simulink model "scattering_pos_pos"  (R2022b)
settings: Solver=VariableStepAuto  StartTime=0.0  StopTime=10.0  RelTol=1e-3
values from neighbouring files (symbols this model uses):
  A = 2    [scattering_params.m]    (also in scattering_params_force_pos.m = 3; scattering_params_pos_pos.m = 1)
  b = 1    [scattering_params.m]    (also in scattering_params_force_pos.m = 40; scattering_params_pos_pos.m = 100)
  Be = 100    [scattering_params.m]    (also in scattering_params_force_pos.m; scattering_params_pos_pos.m)
  Bh = 1.5    [scattering_params.m]    (also in scattering_params_force_pos.m = 1; scattering_params_pos_pos.m = 1)
  Bm = 20*0.8    (= 16)    [scattering_params.m]
  Bs = 80    [scattering_params.m]    (also in scattering_params_force_pos.m = 10)
  Dh = 0.1    [scattering_params.m]    (also in scattering_params_force_pos.m = 16; scattering_params_pos_pos.m = 16)
  Dm = 0    [scattering_params.m]    (also in scattering_params_force_pos.m; scattering_params_pos_pos.m)
  Ds = 0    [scattering_params.m]    (also in scattering_params_force_pos.m; scattering_params_pos_pos.m)
  Fc = 1    [scattering_params.m]    (also in scattering_params_force_pos.m = 0.25; scattering_params_pos_pos.m = 0.25)
  Flp = 5    [scattering_params.m]    (also in scattering_params_force_pos.m = 0.5; scattering_params_pos_pos.m = 0.5)
  Jh = 1    [scattering_params.m]    (also in scattering_params_force_pos.m; scattering_params_pos_pos.m)
  Ke = 200    [scattering_params.m]    (also in scattering_params_force_pos.m; scattering_params_pos_pos.m)
  Km = 10*1    (= 10)    [scattering_params.m]
  Ks = 100    [scattering_params.m]    (also in scattering_params_force_pos.m)
  Mm = 0.5    [scattering_params.m]    (also in scattering_params_force_pos.m; scattering_params_pos_pos.m)
  Ms = 2    [scattering_params.m]    (also in scattering_params_force_pos.m; scattering_params_pos_pos.m)
  Ph = 10    [scattering_params.m]    (also in scattering_params_force_pos.m; scattering_params_pos_pos.m)
  time_delay = 0    [scattering_params.m]
  xe = 5    [scattering_params.m]    (also in scattering_params_force_pos.m = 2; scattering_params_pos_pos.m = 2)
settings Model: Creator=Manu  LastModifiedBy=Manu

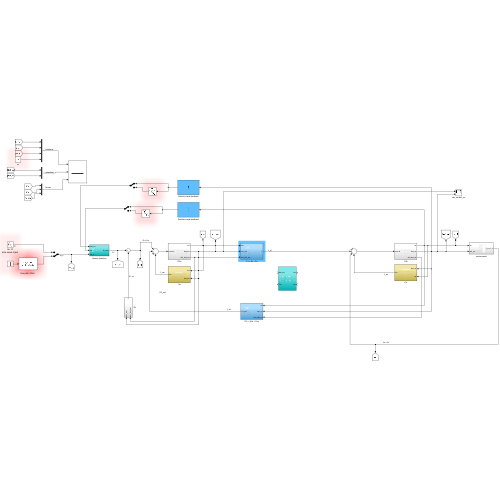
[thumbnail: Simulink's stored preview of the top-level diagram]
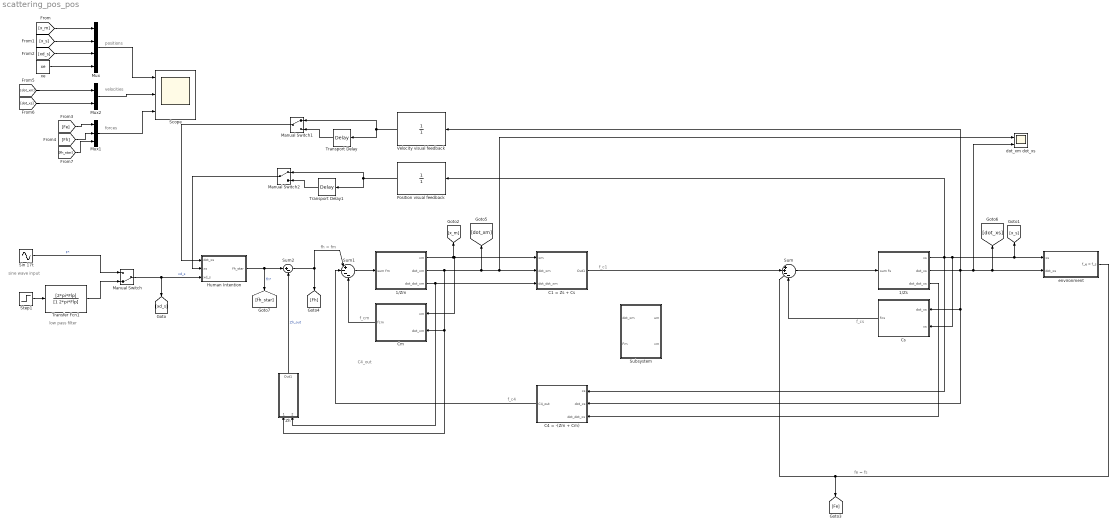
== system scattering_pos_pos ==
  note: positions
  note: fe = fs
  note: C4_out
  note: f_cm
  note: fh = fm
  note: sine wave input
  note: low pass filter
  note: f_cs
  note: forces
  note: velocities
  note: f_c4
  note: f_c1
  1/Zm : Subsystem
  1/Zs : Subsystem
  C1 = Zs + Cs : Subsystem
  C4 = -(Zm + Cm) : Subsystem
  Cm : Subsystem
  Cs : Subsystem
  Human Intention : Subsystem
  Manual Switch : ManualSwitch  CurrentSetting=0
  Manual Switch1 : ManualSwitch
  Manual Switch2 : ManualSwitch
  Mux : Mux
  Mux1 : Mux  Inputs=3
  Mux2 : Mux  Inputs=2
  Position visual feedback : TransferFcn  Denominator=[1]
  Scope : Scope  NumInputPorts=3
  Sin 17t : Sin  Amplitude=A  Frequency=2*pi*Fc  SampleTime=0
  Step1 : Step  Time=0.5  After=A  SampleTime=0
  Subsystem : Subsystem
      settings: PortSchema="{\"entries\":[{\"content\":{\"sides\":[{\"content\":{\"connectorIds\":[\"In1\",\"Out2\"]},\"type\":\"ConnectorPlacement.EquallySpacedRectSide\",\"uuid\":\"82be490b-f4e1-4469-8bd6-488a0e070f91\"},{\"content\":{\"connectorIds\":[\"Out1\",\"In2\"],\"side\":\"RIGHT\"},\"type\":\"ConnectorPlacement.EquallySpacedRectSide\",\"uuid\":\"c4a13bf6-21c5-475e-be70-cb3636e820b8\"},{\"content\":{\"connectorIds\":[],\"side\":\"TOP\"},\"type\":\"ConnectorPlacement.EquallySpacedRectSide\",\"uuid\":\"239945ea-98d9-43ca-9337-d0acd489fa2c\"},{\"content\":{\"connectorIds\":[],\"side\":\"BOTTOM\"},\"type\":\"ConnectorPlacement.EquallySpacedRectSide\",\"uuid\":\"d302d15a-ee16-4e35-85d1-74674ea2a331\"},{\"content\":{\"connectorIds\":[],\"side\":\"HIDDEN\"},\"type\":\"ConnectorPlacement.EquallySpacedRectSide\",\"uuid\":\"ab55d6c9-2d6b-496a-b62d-f74546630c92\"}]},\"type\":\"ConnectorPlacement.EquallySpacedConnector\",\"uuid\":\"f2ee4140-76ed-4153-9f7f-3580e67d072a\"}],\"packageUris\":[\"http://schema.mathworks.com/mf0/Connector/R2020b\"],\"version\":\"1.0\"}"
  Sum : Sum  Inputs=|++--
  Sum1 : Sum  Inputs=|+---
  Sum2 : Sum  Inputs=|+-
  Transfer Fcn1 : TransferFcn  Numerator=[2*pi*Flp]  Denominator=[1 2*pi*Flp]
  Transport Delay : TransportDelay  DelayTime=time_delay
  Transport Delay1 : TransportDelay  DelayTime=time_delay
  Velocity visual feedback : TransferFcn  Denominator=[1]
  Zh : Subsystem
  dot_xm dot_xs : Scope  NumInputPorts=2
  environment : Subsystem
  xe : Constant  Value=xe
  wires:
  1/Zm/2(dot_xm) -> C1 = Zs + Cs/2(dot_xm), dot_xm dot_xs/1, [dot_xm], Cm/2(dot_xm), Zh/1(dot_xm)
  1/Zm/1(xm) -> C1 = Zs + Cs/1(xm), Cm/1(xm), [x_m]
  Manual Switch/1 -> [xd_s], Human Intention/3(xd_s)  "xd_s"
  Zh/1(Out1) -> Sum2/2  "Zh_out"
  Sin 17t/1 -> Manual Switch/1  "F*"
  1/Zm/3(dot_dot_xm) -> C1 = Zs + Cs/3(dot_dot_xm), Zh/2(dot_dot_xm)
  Human Intention/1(fh_star) -> Sum2/1, [fh_star]  "fh*"
  Transfer Fcn1/1 -> Manual Switch/2
  Step1/1 -> Transfer Fcn1/1
  Sum2/1 -> Sum1/1, [Fh]
  Sum1/1 -> 1/Zm/1(sum fm)
  C4 = -(Zm + Cm)/1(C4_out) -> Sum1/2
  C1 = Zs + Cs/1(Out1) -> Sum/2
  Cs/1(fcs) -> Sum/4
  Sum/1 -> 1/Zs/1(sum fs)
  1/Zs/2(dot_xs) -> Velocity visual feedback/1, C4 = -(Zm + Cm)/2(dot_xs), Cs/1(dot_xs), dot_xm dot_xs/2, [dot_xs], environment/2(dot_xs)
  1/Zs/1(xs) -> C4 = -(Zm + Cm)/1(xs), Cs/2(xs), [x_s], environment/1(xs), Position visual feedback/1
  1/Zs/3(dot_dot_xs) -> C4 = -(Zm + Cm)/3(dot_dot_xs)
  environment/1(f_e = f_s) -> Sum/3, [Fe]
  Cm/1(fcm) -> Sum1/4
  Mux/1 -> Scope/1
  [x_s] -> Mux/2
  [xd_s] -> Mux/3
  xe/1 -> Mux/4
  [x_m] -> Mux/1
  Mux1/1 -> Scope/3
  [Fe] -> Mux1/1
  [Fh] -> Mux1/2
  [dot_xs] -> Mux2/2
  [dot_xm] -> Mux2/1
  Mux2/1 -> Scope/2
  [fh_star] -> Mux1/3
  Velocity visual feedback/1 -> Transport Delay/1, Manual Switch1/1
  Transport Delay/1 -> Manual Switch1/2
  Manual Switch1/1 -> Human Intention/1(dot_xs)
  Transport Delay1/1 -> Manual Switch2/2
  Position visual feedback/1 -> Transport Delay1/1, Manual Switch2/1
  Manual Switch2/1 -> Human Intention/2(xs)

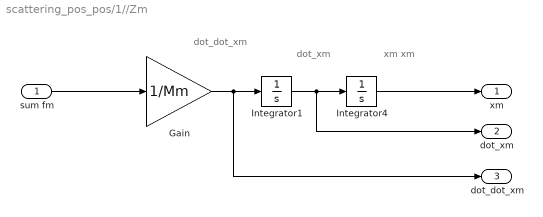
== system scattering_pos_pos/1//Zm ==
  note: dot_dot_xm
  note: dot_xm
  note: xm
      | xm
  sum fm : Inport
  Gain : Gain  Gain=1/Mm
  Integrator1 : Integrator
  Integrator4 : Integrator
  xm : Outport
  dot_xm : Outport  Port=2
  dot_dot_xm : Outport  Port=3
  wires:
  sum fm/1 -> Gain/1
  Gain/1 -> dot_dot_xm/1, Integrator1/1
  Integrator4/1 -> xm/1
  Integrator1/1 -> dot_xm/1, Integrator4/1

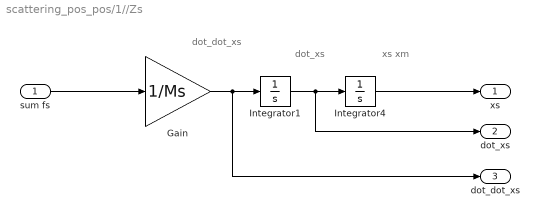
== system scattering_pos_pos/1//Zs ==
  note: dot_dot_xs
  note: dot_xs
  note: xs
      | xm
  sum fs : Inport
  Gain : Gain  Gain=1/Ms
  Integrator1 : Integrator
  Integrator4 : Integrator
  xs : Outport
  dot_xs : Outport  Port=2
  dot_dot_xs : Outport  Port=3
  wires:
  sum fs/1 -> Gain/1
  Gain/1 -> dot_dot_xs/1, Integrator1/1
  Integrator4/1 -> xs/1
  Integrator1/1 -> dot_xs/1, Integrator4/1

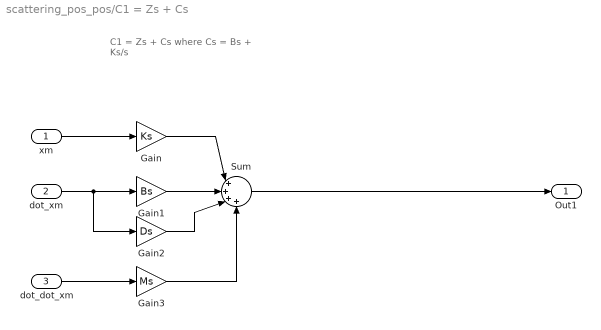
== system scattering_pos_pos/C1 = Zs + Cs ==
  note: C1 = Zs + Cs
      | where
      | Cs = Bs + Ks/s
  xm : Inport
  dot_xm : Inport  Port=2
  dot_dot_xm : Inport  Port=3
  Gain : Gain  Gain=Ks
  Gain1 : Gain  Gain=Bs
  Gain2 : Gain  Gain=Ds
  Gain3 : Gain  Gain=Ms
  Sum : Sum  Inputs=|++++
  Out1 : Outport
  wires:
  xm/1 -> Gain/1
  Gain/1 -> Sum/1
  dot_xm/1 -> Gain2/1, Gain1/1
  Gain1/1 -> Sum/2
  Gain2/1 -> Sum/3
  dot_dot_xm/1 -> Gain3/1
  Gain3/1 -> Sum/4
  Sum/1 -> Out1/1

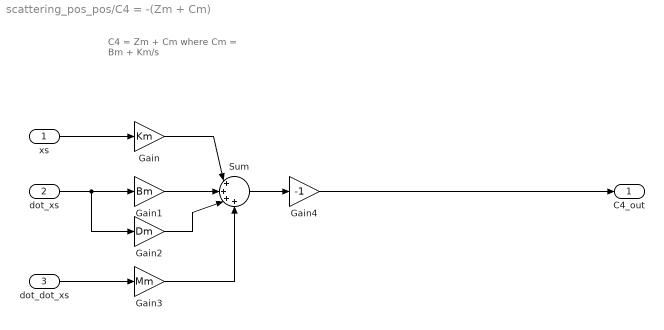
== system scattering_pos_pos/C4 = -(Zm + Cm) ==
  note: C4 = Zm + Cm
      | where
      | Cm = Bm + Km/s
  xs : Inport
  dot_xs : Inport  Port=2
  dot_dot_xs : Inport  Port=3
  Gain : Gain  Gain=Km
  Gain1 : Gain  Gain=Bm
  Gain2 : Gain  Gain=Dm
  Gain3 : Gain  Gain=Mm
  Gain4 : Gain  Gain=-1
  Sum : Sum  Inputs=|++++
  C4_out : Outport
  wires:
  xs/1 -> Gain/1
  Gain/1 -> Sum/1
  dot_xs/1 -> Gain2/1, Gain1/1
  Gain1/1 -> Sum/2
  Gain2/1 -> Sum/3
  dot_dot_xs/1 -> Gain3/1
  Gain3/1 -> Sum/4
  Sum/1 -> Gain4/1
  Gain4/1 -> C4_out/1

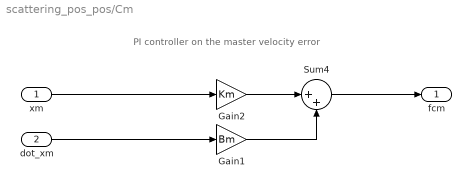
== system scattering_pos_pos/Cm ==
  note: PI controller on the master velocity error
  xm : Inport
  dot_xm : Inport  Port=2
  Gain1 : Gain  Gain=Bm
  Gain2 : Gain  Gain=Km
  Sum4 : Sum  Inputs=|++
  fcm : Outport
  wires:
  Sum4/1 -> fcm/1
  xm/1 -> Gain2/1
  Gain2/1 -> Sum4/1
  dot_xm/1 -> Gain1/1
  Gain1/1 -> Sum4/2

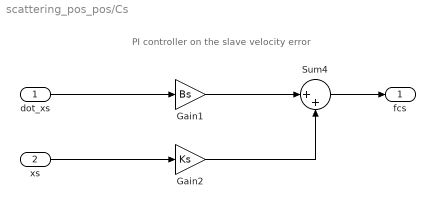
== system scattering_pos_pos/Cs ==
  note: PI controller on the slave velocity error
  dot_xs : Inport
  xs : Inport  Port=2
  Gain1 : Gain  Gain=Bs
  Gain2 : Gain  Gain=Ks
  Sum4 : Sum  Inputs=|++
  fcs : Outport
  wires:
  Sum4/1 -> fcs/1
  xs/1 -> Gain2/1
  Gain2/1 -> Sum4/2
  dot_xs/1 -> Gain1/1
  Gain1/1 -> Sum4/1

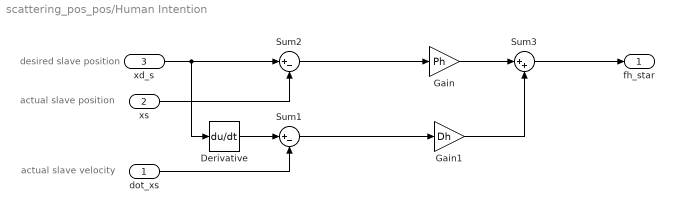
== system scattering_pos_pos/Human Intention ==
  note: actual slave velocity
  note: actual slave position
  note: desired slave position
  dot_xs : Inport
  xs : Inport  Port=2
  xd_s : Inport  Port=3
  Derivative : Derivative
  Gain : Gain  Gain=Ph
  Gain1 : Gain  Gain=Dh
  Sum1 : Sum  Inputs=|+-
  Sum2 : Sum  Inputs=|+-
  Sum3 : Sum  Inputs=|++
  fh_star : Outport
  wires:
  xs/1 -> Sum2/2
  dot_xs/1 -> Sum1/2
  Sum2/1 -> Gain/1
  Sum1/1 -> Gain1/1
  Gain1/1 -> Sum3/2
  Gain/1 -> Sum3/1
  Sum3/1 -> fh_star/1
  xd_s/1 -> Derivative/1, Sum2/1
  Derivative/1 -> Sum1/1

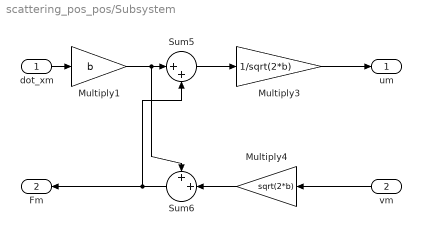
== system scattering_pos_pos/Subsystem ==
  dot_xm : Inport
  vm : Inport  Port=2
  Multiply1 : Gain  Gain=b
  Multiply3 : Gain  Gain=1/sqrt(2*b)
  Multiply4 : Gain  Gain=sqrt(2*b)
  Sum5 : Sum  Inputs=|++
  Sum6 : Sum  Inputs=++|
  um : Outport
  Fm : Outport  Port=2
  wires:
  Sum6/1 -> Fm/1, Sum5/2
  Multiply1/1 -> Sum6/1, Sum5/1
  Sum5/1 -> Multiply3/1
  Multiply4/1 -> Sum6/2
  vm/1 -> Multiply4/1
  Multiply3/1 -> um/1
  dot_xm/1 -> Multiply1/1

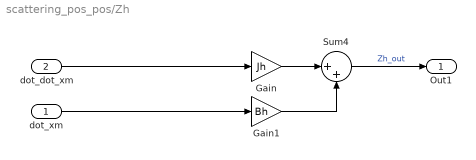
== system scattering_pos_pos/Zh ==
  dot_xm : Inport
  dot_dot_xm : Inport  Port=2
  Gain : Gain  Gain=Jh
  Gain1 : Gain  Gain=Bh
  Sum4 : Sum  Inputs=|++
  Out1 : Outport
  wires:
  dot_dot_xm/1 -> Gain/1
  Gain1/1 -> Sum4/2
  Gain/1 -> Sum4/1
  Sum4/1 -> Out1/1  "Zh_out"
  dot_xm/1 -> Gain1/1

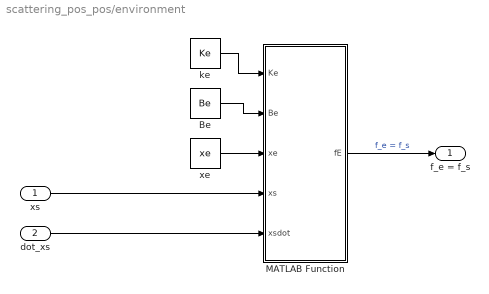
== system scattering_pos_pos/environment ==
  xs : Inport
  dot_xs : Inport  Port=2
  Be : Constant  Value=Be
  MATLAB Function : MATLAB Function  TreatAsAtomicUnit=on
  ke : Constant  Value=Ke
  xe : Constant  Value=xe
  f_e = f_s : Outport
  wires:
  MATLAB Function/1(fE) -> f_e = f_s/1  "f_e = f_s"
  xs/1 -> MATLAB Function/4(xs)
  xe/1 -> MATLAB Function/3(xe)
  dot_xs/1 -> MATLAB Function/5(xsdot)
  ke/1 -> MATLAB Function/1(Ke)
  Be/1 -> MATLAB Function/2(Be)

== matlab function scattering_pos_pos/environment/MATLAB Function ==
  data: Ke input; fE output; Be input; xe input; xs input; xsdot input
function fE = environment(Ke, Be, xe, xs, xsdot)
    if xs > xe
        fE = Ke * (xs - xe) + Be * xsdot; % Plot both contributions Ke and Be
    else
        fE = 0;
    end
end
